simulink model "slproject_f14"  (R2015a)
settings: Solver=ode45  StartTime=0.0  StopTime=10.0  MaxStep=0.1  RelTol=1e-3
undefined symbols (not defined in the file): g, Uo
libraries: wind_gust_lib x1
settings Model: ModifiedByFormat=The MathWorks Inc.  CovSFcnEnable=off  Creator=The MathWorks Inc.  LastModifiedBy=The MathWorks Inc.
settings ConfigSet: ConfigType=Model
settings SolverCC: Priority=auto
settings DataIOCC: SaveOutput=off  SaveTime=off  SignalLoggingName=slproject_f14
settings OptimizationCC: InlineParamsCompatibleMode=off  ExpressionDepthLimit=2147483647  InitFltsAndDblsToZero=on  ForceBlockIOInitOptimize=off  EvaledLifeSpan=1  SimCompilerOptimization=Off
settings DebuggingCC: SaveWithParameterizedLinksMsg=none  UnderspecifiedInitializationDetection=Classic  MergeDetectMultiDrivingBlocksExec=none  SignalResolutionControl=TryResolveAllWithWarning  SolverPrmCheckMsg=warning  MultiTaskDSMMsg=warning  MultiTaskCondExecSysMsg=none  FcnCallInpInsideContextMsg=UseLocalSettings  AllowSymbolicDim=off  StateNameClashWarn=warning  SFMismatchInSimAndRtwBecauseOfMissingDataTypeDiag=warning
settings ModelReferenceCC: ModelReferenceMinAlgLoopOccurrences=on
settings RTWCC: EnableTagging=off  RTWCompilerOptimization=Off
settings CodeAppCC: ParameterTuningSideEffectCode=Output function  AllmanStyle=off
settings GRTTargetCC: TargetFcnLib=ansi_tfl_tmw.mat  CombineOutputUpdateFcns=off  EnableShiftOperators=off  PortableWordSizesTransition=off  GenerateErtSFunctionTransition=off  CreateSILPILBlockTransition=None  CodeProfilingSaveOptionsTransition=SummaryOnly  CodeExecutionProfilingTransition=off  CodeProfilingInstrumentationTransition=off  CodeExecutionProfileVariableTransition=executionProfile  GRTInterface=on

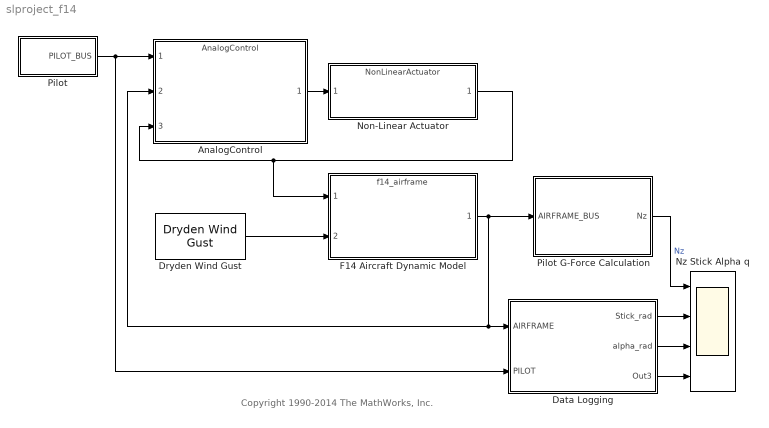
== system slproject_f14 ==
  note: Copyright 1990-2014 The MathWorks, Inc.
  AnalogControl : ModelReference  IOType=none  Commented=off  StatePerturbationForJacobian=1.0e-05  ModelNameDialog=AnalogControl  SimulationMode=Normal  ModelReferenceVersion=1.21  CopyOfModelName=AnalogControl  DefaultDataLogging=on
  Data Logging : Subsystem  IOType=none  Commented=off  StatePerturbationForJacobian=1.0e-05
  Dryden Wind Gust : wind_gust_lib/Dryden Wind Gust  IOType=none  Commented=off  StatePerturbationForJacobian=1.0e-05
  F14 Aircraft Dynamic Model : ModelReference  IOType=none  Commented=off  StatePerturbationForJacobian=1.0e-05  ModelNameDialog=f14_airframe  SimulationMode=Normal  ModelReferenceVersion=1.25  CopyOfModelName=f14_airframe  DefaultDataLogging=on
  Non-Linear Actuator : ModelReference  IOType=none  Commented=off  StatePerturbationForJacobian=1.0e-05  ModelNameDialog=NonLinearActuator  SimulationMode=Normal  ModelReferenceVersion=1.27  CopyOfModelName=NonLinearActuator  DefaultDataLogging=on
  Nz Stick Alpha q : Scope  Commented=off  NumInputPorts=4
      settings: IOType=none  StatePerturbationForJacobian=1.0e-05  TickLabels=on  TimeRange=15  YMin=-1~-1.5~-3~-15  YMax=1~1.5~3~15
  Pilot : Subsystem  IOType=none  Commented=off  StatePerturbationForJacobian=1.0e-05
  Pilot G-Force Calculation : Subsystem  IOType=none  Commented=off  StatePerturbationForJacobian=1.0e-05
  wires:
  Pilot/1(PILOT_BUS) -> Data Logging/2(PILOT), AnalogControl/1
  F14 Aircraft Dynamic Model/1 -> Pilot G-Force Calculation/1(AIRFRAME_BUS), AnalogControl/2, Data Logging/1(AIRFRAME)
  Dryden Wind Gust/1 -> F14 Aircraft Dynamic Model/2
  Pilot G-Force Calculation/1(Nz) -> Nz Stick Alpha q/1  "Nz"
  Data Logging/1(Stick_rad) -> Nz Stick Alpha q/2
  Data Logging/2(alpha_rad) -> Nz Stick Alpha q/3
  Data Logging/3(Out3) -> Nz Stick Alpha q/4
  AnalogControl/1 -> Non-Linear Actuator/1
  Non-Linear Actuator/1 -> AnalogControl/3, F14 Aircraft Dynamic Model/1

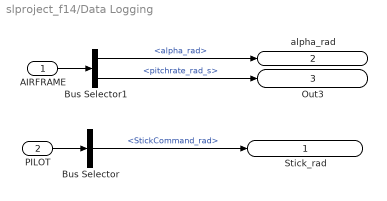
== system slproject_f14/Data Logging ==
  AIRFRAME : Inport  IOType=none  Commented=off  StatePerturbationForJacobian=1.0e-05
  PILOT : Inport  IOType=none  Commented=off  StatePerturbationForJacobian=1.0e-05  Port=2
  Bus Selector : BusSelector  IOType=none  Commented=off  StatePerturbationForJacobian=1.0e-05  OutputSignals=StickCommand_rad
  Bus Selector1 : BusSelector  IOType=none  Commented=off  StatePerturbationForJacobian=1.0e-05  OutputSignals=alpha_rad,pitchrate_rad_s
  Stick_rad : Outport  IOType=none  Commented=off  StatePerturbationForJacobian=1.0e-05
  alpha_rad : Outport  IOType=none  Commented=off  StatePerturbationForJacobian=1.0e-05  Port=2
  Out3 : Outport  IOType=none  Commented=off  StatePerturbationForJacobian=1.0e-05  Port=3
  wires:
  PILOT/1 -> Bus Selector/1
  AIRFRAME/1 -> Bus Selector1/1
  Bus Selector/1 -> Stick_rad/1  "<StickCommand_rad>"
  Bus Selector1/1 -> alpha_rad/1  "<alpha_rad>"
  Bus Selector1/2 -> Out3/1  "<pitchrate_rad_s>"

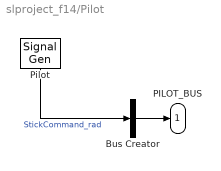
== system slproject_f14/Pilot ==
  Bus Creator : BusCreator  IOType=none  Commented=off  StatePerturbationForJacobian=1.0e-05  Inputs=1  OutDataTypeStr=Bus: PILOT_BUS
  Pilot : SignalGenerator  IOType=none  Commented=off  StatePerturbationForJacobian=1.0e-05  WaveForm=square  Frequency=.1
  PILOT_BUS : Outport  IOType=none  Commented=off  StatePerturbationForJacobian=1.0e-05  OutDataTypeStr=Bus: PILOT_BUS
  wires:
  Pilot/1 -> Bus Creator/1  "StickCommand_rad"
  Bus Creator/1 -> PILOT_BUS/1

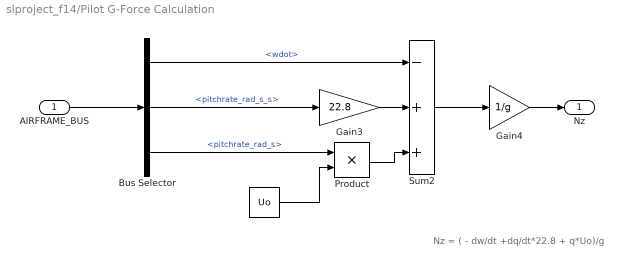
== system slproject_f14/Pilot G-Force Calculation ==
  note: Nz = ( - dw/dt +dq/dt*22.8 + q*Uo)/g
  AIRFRAME_BUS : Inport  IOType=none  Commented=off  StatePerturbationForJacobian=1.0e-05
  " " : Constant  IOType=none  Commented=off  StatePerturbationForJacobian=1.0e-05  Value=Uo
  Bus Selector : BusSelector  IOType=none  Commented=off  StatePerturbationForJacobian=1.0e-05  OutputSignals=wdot,pitchrate_rad_s_s,pitchrate_rad_s
  Gain3 : Gain  IOType=none  Commented=off  StatePerturbationForJacobian=1.0e-05  Gain=22.8  SaturateOnIntegerOverflow=on  OutDataTypeStr=Inherit: Same as input  ParamDataTypeStr=Inherit: Same as input
  Gain4 : Gain  IOType=none  Commented=off  StatePerturbationForJacobian=1.0e-05  Gain=1/g  SaturateOnIntegerOverflow=on  OutDataTypeStr=Inherit: Same as input  ParamDataTypeStr=Inherit: Same as input
  Product : Product  IOType=none  Commented=off  StatePerturbationForJacobian=1.0e-05  SaturateOnIntegerOverflow=on  RndMeth=Zero  InputSameDT=on  OutDataTypeStr=Inherit: Same as first input
  Sum2 : Sum  IOType=none  Commented=off  StatePerturbationForJacobian=1.0e-05  Inputs=-++  SaturateOnIntegerOverflow=on  InputSameDT=on  OutDataTypeStr=Inherit: Same as first input
  Nz : Outport  IOType=none  Commented=off  StatePerturbationForJacobian=1.0e-05
  wires:
  " "/1 -> Product/2
  Bus Selector/3 -> Product/1  "<pitchrate_rad_s>"
  Product/1 -> Sum2/3
  Gain3/1 -> Sum2/2
  Bus Selector/2 -> Gain3/1  "<pitchrate_rad_s_s>"
  Gain4/1 -> Nz/1
  Bus Selector/1 -> Sum2/1  "<wdot>"
  Sum2/1 -> Gain4/1
  AIRFRAME_BUS/1 -> Bus Selector/1
